simulink model "UAV_log"  (R2019b)
settings: Solver=FixedStepAuto  StartTime=0.0  StopTime=100  RelTol=1e-3
InitFcn:
  | load('BusDefinitions.mat')
values from neighbouring files (symbols this model uses):
  A_double = [0 1; 0 0]    [kalman_matrices_calculator.m]
  A_s_double = eval(subs(Ad_double,Ts))    [kalman_matrices_calculator.m]
  A_s_single = eval(subs(Ad_single,Ts))    [kalman_matrices_calculator.m]
  A_single = [0]    [kalman_matrices_calculator.m]
  B_double = [0; 1]    [kalman_matrices_calculator.m]
  B_s_double = eval(subs(Bd_double,Ts))    [kalman_matrices_calculator.m]
  B_s_single = eval(subs(Bd_single,Ts))    [kalman_matrices_calculator.m]
  B_single = [1]    [kalman_matrices_calculator.m]
  C_double = [1 0]    [kalman_matrices_calculator.m]
  C_single = [1]    [kalman_matrices_calculator.m]
  D_double = [0]    [kalman_matrices_calculator.m]
  D_single = [0]    [kalman_matrices_calculator.m]
  L_double = lqe(A_double, G_double, C_double, q_double, r_double, 0)    [kalman_matrices_calculator.m]
  L_single = lqe(A_single, G_single, C_single, q_single, r_single, 0)    [kalman_matrices_calculator.m]
  q_single = cov(out.In_Out_Data{1}.Values.Data)    [kalman_matrices_calculator.m]
  r_single = cov(out.In_Out_Data{2}.Values.Data)    [kalman_matrices_calculator.m]
  Ts = 0.005    [kalman_matrices_calculator.m]
undefined symbols (not defined in the file or in its folder): codertarget, DiscIntNeverNeededParam, Discrete, Time
libraries: ctrlSharedLib x5
settings Model: ExtModeTrigDuration=80  Creator=Sankalp Bhan  LastModifiedBy=Chris
settings OptimizationCC: PassReuseOutputArgsThreshold=0  MaxStackSize=64
settings DebuggingCC: ParameterTunabilityLossMsg=error  ArithmeticOperatorsInVariantConditions=warning
settings HardwareCC: ProdBitPerPointer=32  ProdBitPerSizeT=32  ProdBitPerPtrDiffT=32  ProdLargestAtomicInteger=Long  ProdWordSize=32  ProdHWDeviceType=ARM Compatible->ARM 9  UseEmbeddedCoderFeatures=off
settings SFSimCC: SimUseLocalCustomCode=off  MATLABDynamicMemAlloc=off
settings RTWCC: SystemTargetFile=ert.tlc  HardwareBoard=PARROT Mambo  TLCOptions="-aInlineSetEventsForThisBaseRateFcn=TLC_FALSE -aSuppressMultiTaskScheduler=TLC_FALSE   -aRateBasedStepFcn=1"  TemplateMakefile=ert_default_tmf  GenerateReport=on  RTWUseLocalCustomCode=off  Toolchain=Sourcery G++ Lite GNU Toolchain for Drones  LaunchReport=on
settings CodeAppCC: ForceParamTrailComments=on  OperatorAnnotations=on  StateflowObjectComments=on
settings ERTTargetCC: ERTCustomFileBanners=off  MatFileLogging=on  SupportContinuousTime=on  SupportNonInlinedSFcns=on  RemoveResetFunc=off  ModelStepFunctionPrototypeControlCompliant=off

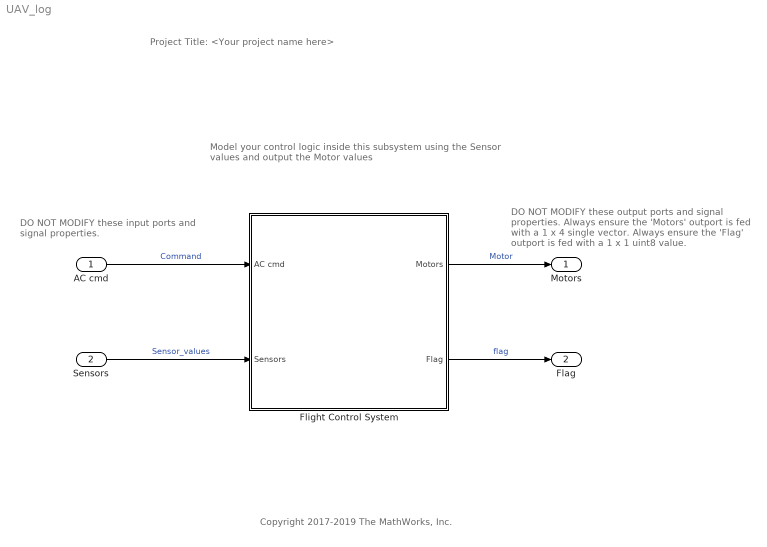
== system UAV_log ==
  note: Model your control logic inside this subsystem
      | using the Sensor values and output the
      | Motor values
  note: DO NOT MODIFY these output ports
      | and signal properties.
      |
      |
      |
      | Always ensure the 'Motors' outport
      | is fed with a 1 x 4 single vector.
      |
      |
      |
      |
      |
      | Always ensure the 'Flag' outport is
      | fed with a 1 x 1 uint8 value.
  note: DO NOT MODIFY these input
      | ports and signal properties.
  note: Copyright 2017-2019 The MathWorks, Inc.
  note: Project Title: <Your project name here>
  AC cmd : Inport  OutDataTypeStr=Bus: CommandBus  BusOutputAsStruct=on
  Sensors : Inport  Port=2  OutDataTypeStr=Bus: SensorsBus  BusOutputAsStruct=on
  Flight Control System : Subsystem  InitFcn=codertarget.parrot.internal.fcsSubsystemCallback(gcb);
  Motors : Outport  OutDataTypeStr=single  PortDimensions=[1 4]  VectorParamsAs1DForOutWhenUnconnected=off
  Flag : Outport  Port=2  OutDataTypeStr=uint8  PortDimensions=1  VectorParamsAs1DForOutWhenUnconnected=off
  wires:
  Flight Control System/1(Motors) -> Motors/1  "Motor"
  AC cmd/1 -> Flight Control System/1(AC cmd)  "Command"
  Sensors/1 -> Flight Control System/2(Sensors)  "Sensor_values"
  Flight Control System/2(Flag) -> Flag/1  "flag"

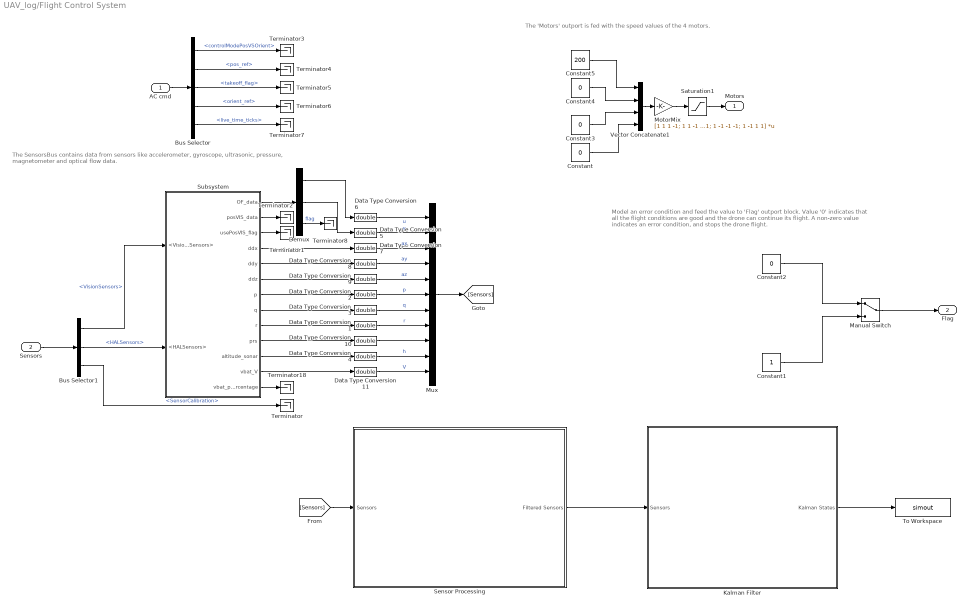
== system UAV_log/Flight Control System ==
  note: The 'Motors' outport is fed with the speed values of the 4 motors.
  note: Model an error condition and feed the value to 'Flag' outport block.
      | Value '0' indicates that all the flight conditions are good and the drone
      | can continue its flight.
      | A non-zero value indicates an error condition, and stops the drone
      | flight.
  note: The SensorsBus contains data from sensors like
      | accelerometer, gyroscope, ultrasonic, pressure,
      | magnetometer and optical flow data.
  AC cmd : Inport
  Sensors : Inport  Port=2
  Bus Selector : BusSelector  OutputSignals=controlModePosVSOrient,pos_ref,takeoff_flag,orient_ref,live_time_ticks
  Bus Selector1 : BusSelector  OutputSignals=VisionSensors,HALSensors,SensorCalibration
  Constant : Constant  Value=0  SampleTime=Ts
  Constant1 : Constant  OutDataTypeStr=uint8
  Constant2 : Constant  Value=0  OutDataTypeStr=uint8
  Constant3 : Constant  Value=0  SampleTime=Ts
  Constant4 : Constant  Value=0  SampleTime=Ts
  Constant5 : Constant  Value=200  SampleTime=Ts
  Data Type Conversion{1..11} (11 alike) : DataTypeConversion  OutDataTypeStr=double
  Demux : Demux  Outputs=3
  Kalman Filter : Subsystem
  Manual Switch : ManualSwitch
  MotorMix : Gain  Gain=[1 1 1 -1; 1 1 -1 1; 1 -1 -1 -1; 1 -1 1 1]  Multiplication=Matrix(K*u)
  Mux : Mux  Inputs=11
  Saturation1 : Saturate  UpperLimit=500  LowerLimit=0  OutDataTypeStr=single
  "Sensor Processing " : Subsystem
  Subsystem : Subsystem
  Terminator{,1..8,18} (10 alike) : Terminator
  To Workspace : ToWorkspace  VariableName=simout  SaveFormat=Structure With Time  SampleTime=-1
  Vector Concatenate1 : Concatenate  NumInputs=4
  Motors : Outport  VectorParamsAs1DForOutWhenUnconnected=off
  Flag : Outport  Port=2  VectorParamsAs1DForOutWhenUnconnected=off
  wires:
  AC cmd/1 -> Bus Selector/1
  Sensors/1 -> Bus Selector1/1
  Bus Selector/1 -> Terminator3/1  "<controlModePosVSOrient>"
  Bus Selector/2 -> Terminator4/1  "<pos_ref>"
  Bus Selector/3 -> Terminator5/1  "<takeoff_flag>"
  Bus Selector/4 -> Terminator6/1  "<orient_ref>"
  Bus Selector/5 -> Terminator7/1  "<live_time_ticks>"
  Manual Switch/1 -> Flag/1
  Constant2/1 -> Manual Switch/1
  Constant1/1 -> Manual Switch/2
  Vector Concatenate1/1 -> MotorMix/1
  Constant5/1 -> Vector Concatenate1/1
  Constant/1 -> Vector Concatenate1/4
  Constant4/1 -> Vector Concatenate1/2
  Constant3/1 -> Vector Concatenate1/3
  Saturation1/1 -> Motors/1
  Bus Selector1/1 -> Subsystem/1(<VisionSensors>)  "<VisionSensors>"
  Bus Selector1/2 -> Subsystem/2(<HALSensors>)  "<HALSensors>"
  Bus Selector1/3 -> Terminator/1  "<SensorCalibration>"
  Subsystem/1(OF_data) -> Demux/1
  Subsystem/4(ddx) -> Data Type Conversion7/1
  Subsystem/5(ddy) -> Data Type Conversion8/1
  Subsystem/6(ddz) -> Data Type Conversion9/1
  Subsystem/7(p) -> Data Type Conversion2/1
  Subsystem/9(r) -> Data Type Conversion1/1
  Subsystem/11(altitude_sonar) -> Data Type Conversion4/1
  Subsystem/12(vbat_V) -> Data Type Conversion11/1
  Subsystem/13(vbat_percentage) -> Terminator18/1
  Subsystem/8(q) -> Data Type Conversion3/1
  Mux/1 -> [Sensors]
  MotorMix/1 -> Saturation1/1
  Subsystem/3(usePosVIS_flag) -> Terminator1/1
  Subsystem/2(posVIS_data) -> Terminator2/1
  Demux/1 -> Data Type Conversion6/1
  Demux/2 -> Data Type Conversion5/1
  Demux/3 -> Terminator8/1  "flag"
  Subsystem/10(prs) -> Data Type Conversion10/1
  Data Type Conversion1/1 -> Mux/8  "r"
  Data Type Conversion2/1 -> Mux/6  "p"
  Data Type Conversion3/1 -> Mux/7  "q"
  Data Type Conversion4/1 -> Mux/10  "h"
  Data Type Conversion5/1 -> Mux/2  "v"
  Data Type Conversion6/1 -> Mux/1  "u"
  Data Type Conversion7/1 -> Mux/3  "ax"
  Data Type Conversion8/1 -> Mux/4  "ay"
  Data Type Conversion9/1 -> Mux/5  "az"
  Data Type Conversion10/1 -> Mux/9
  Data Type Conversion11/1 -> Mux/11  "V"
  [Sensors] -> "Sensor Processing "/1(Sensors)
  "Sensor Processing "/1(Filtered Sensors) -> Kalman Filter/1(Sensors)
  Kalman Filter/1(Kalman States) -> To Workspace/1

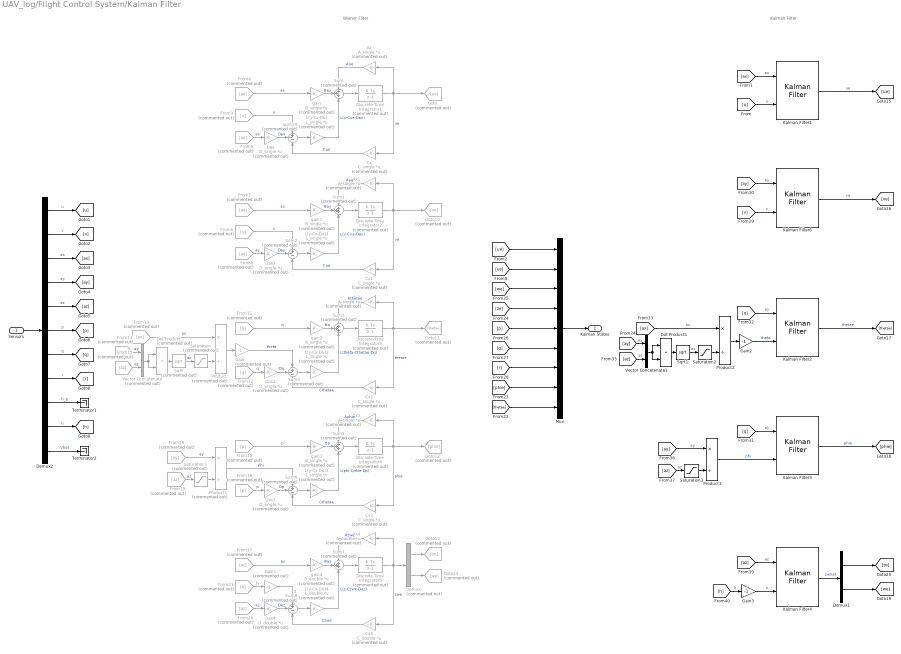
== system UAV_log/Flight Control System/Kalman Filter ==
  note: Wiener Filter
  note: Kalman Filter
  Sensors : Inport
  Ax{,1..3} (4 alike) : Gain  Commented=on  Gain=A_single  Multiplication=Matrix(K*u)
      settings: AttributesFormatString=Ax
  Ax4 : Gain  Commented=on  Gain=A_double  Multiplication=Matrix(K*u)
      settings: AttributesFormatString=Ax
  Cx{,1..3} (4 alike) : Gain  Commented=on  Gain=C_single  Multiplication=Matrix(K*u)
      settings: AttributesFormatString=Cx
  Cx4 : Gain  Commented=on  Gain=C_double  Multiplication=Matrix(K*u)
      settings: AttributesFormatString=Cx
  Dax{,1..3} (4 alike) : Gain  Commented=on  Gain=D_single  Multiplication=Matrix(K*u)
      settings: AttributesFormatString=Du
  Dax4 : Gain  Commented=on  Gain=D_double  Multiplication=Matrix(K*u)
      settings: AttributesFormatString=Du
  Demux : Demux  Commented=on  Outputs=2
  Demux1 : Demux  Outputs=2
  Demux2 : Demux  Outputs=11
  Discrete-Time Integrator{1..5} (5 alike) : DiscreteIntegrator  Commented=on  SampleTime=-1  ICPrevOutput=DiscIntNeverNeededParam  ICPrevScaledInput=DiscIntNeverNeededParam
  Dot Product : DotProduct  Commented=on  OutMin=0.0001  InputSameDT=on  OutDataTypeStr=Inherit: Inherit via internal rule
  Dot Product1 : DotProduct  OutMin=0.0001  InputSameDT=on  OutDataTypeStr=Inherit: Inherit via internal rule
  From10 : From  Commented=on  GotoTag=p
  From11 : From  Commented=on  GotoTag=q
  From12 : From  Commented=on  GotoTag=q
  From13 : From  Commented=on  GotoTag=ax
  From{7..8,14,18} (4 alike) : From  Commented=on  GotoTag=ay
  From{15,17,19..20} (4 alike) : From  Commented=on  GotoTag=az
  From16 : From  Commented=on  GotoTag=p
  From21 : From  Commented=on  GotoTag=h
  From3 : From  Commented=on  GotoTag=u
  From4 : From  Commented=on  GotoTag=ax
  From5 : From  Commented=on  GotoTag=ax
  From6 : From  Commented=on  GotoTag=v
  Gain : Gain  Commented=on  Gain=-1
  Gain1 : Gain  Commented=on  Gain=-1
  Gain2 : Gain  Gain=-1
  Gain3 : Gain  Gain=-1
  Goto : Goto  Commented=on  GotoTag=ue
  Goto10 : Goto  Commented=on  GotoTag=ve
  Goto11 : Goto  Commented=on  GotoTag=thetae
  Goto12 : Goto  Commented=on  GotoTag=phie
  Goto13 : Goto  Commented=on  GotoTag=we
  Goto14 : Goto  Commented=on  GotoTag=ze
  Kalman Filter{1..3,6} (4 alike) : ctrlSharedLib/Kalman Filter  TimeDomain=Discrete-Time  UseCurrentEstimator=on  ModelSource=Individual A, B, C, D matrices  ModelSourceVariable=ss(0.95,1,1,0,1)  A=A_s_single  B=B_s_single  C=C_single  D=D_single  NumberOfStates=1  NumberOfInputs=1  NumberOfOutputs=1  InitialEstimateSource=Dialog  X0=[0]  P0=10  UseK=off  UseGH=off  NumberOfProcessNoiseInputs=1  G=1  TimeInvariantG=on  H=0  TimeInvariantH=on  Q=[1]*q_single  TimeInvariantQ=on  R=[1]*r_single*10000  TimeInvariantR=on  N=0  TimeInvariantN=on  AddInputPort=on  AddEnablePort=off  OutputEstimatedY=off  OutputP=off  Ts=Ts
      settings: SourceProductBaseCode=CT
  Kalman Filter4 : ctrlSharedLib/Kalman Filter  TimeDomain=Discrete-Time  UseCurrentEstimator=on  ModelSource=Individual A, B, C, D matrices  ModelSourceVariable=ss(0.95,1,1,0,1)  A=A_s_double  B=B_s_double  C=C_double  D=D_double  NumberOfStates=1  NumberOfInputs=1  NumberOfOutputs=1  InitialEstimateSource=Dialog  X0=[0]  P0=10  UseK=off  UseGH=off  NumberOfProcessNoiseInputs=1  G=1  TimeInvariantG=on  H=0  TimeInvariantH=on  Q=[1]*q_single  TimeInvariantQ=on  R=[1]*r_single*10000  TimeInvariantR=on  N=0  TimeInvariantN=on  AddInputPort=on  AddEnablePort=off  OutputEstimatedY=off  OutputP=off  Ts=Ts
      settings: SourceProductBaseCode=CT
  L(y-Cx-Du){,1..3} (4 alike) : Gain  Commented=on  Gain=L_single  Multiplication=Matrix(K*u)
      settings: AttributesFormatString=L(y-Cx-Du)
  L(y-Cx-Du)4 : Gain  Commented=on  Gain=L_double  Multiplication=Matrix(K*u)
      settings: AttributesFormatString=L(y-Cx-Du)
  Mux : Mux  Inputs=9
  Product : Product  Commented=on  Inputs=*/
  Product1 : Product  Commented=on  Inputs=*/
  Product2 : Product  Inputs=*/
  Product3 : Product  Inputs=*/
  Saturation : Saturate  Commented=on  UpperLimit=inf  LowerLimit=0.001
  Saturation1 : Saturate  Commented=on  UpperLimit=inf  LowerLimit=0.001
  Saturation2 : Saturate  UpperLimit=inf  LowerLimit=0.001
  Saturation3 : Saturate  UpperLimit=inf  LowerLimit=0.001
  Sqrt : Sqrt  Commented=on  SaturateOnIntegerOverflow=on
  Sqrt1 : Sqrt  SaturateOnIntegerOverflow=on
  Sum{,1,3,5,7} (5 alike) : Sum  Commented=on  Inputs=+++
  Sum{2,4,6,8,10} (5 alike) : Sum  Commented=on  Inputs=+--
  Terminator1 : Terminator
  Terminator2 : Terminator
  Vector Concatenate : Concatenate  Commented=on
  Vector Concatenate1 : Concatenate
  gain{,1..3} (4 alike) : Gain  Commented=on  Gain=B_single  Multiplication=Matrix(K*u)
      settings: AttributesFormatString=Bu
  gain4 : Gain  Commented=on  Gain=B_double  Multiplication=Matrix(K*u)
      settings: AttributesFormatString=Bu
  Kalman States : Outport
  wires:
  Discrete-Time Integrator1/1 -> Goto/1, Cx/1, Ax/1  "ue"
  Sum10/1 -> L(y-Cx-Du)/1
  Ax/1 -> Sum/1  "Aue"
  L(y-Cx-Du)/1 -> Sum/3  "L(u-Cue-Dax)"
  Cx/1 -> Sum10/3  "Cue"
  From4/1 -> gain/1  "ax"
  gain/1 -> Sum/2  "Bax"
  From3/1 -> Sum10/1  "u"
  From5/1 -> Dax/1  "ax"
  Dax/1 -> Sum10/2  "Dax"
  Sum/1 -> Discrete-Time Integrator1/1
  Demux2/9 -> Terminator1/1  "h_p"
  Demux2/1 -> [u]  "u"
  Demux2/4 -> [ay]  "ay"
  Demux2/3 -> [ax]  "ax"
  Sensors/1 -> Demux2/1
  Demux2/2 -> [v]  "v"
  Demux2/10 -> [h]  "h"
  Demux2/5 -> [az]  "az"
  Demux2/7 -> [q]  "q"
  Demux2/8 -> [r]  "r"
  Demux2/6 -> [p]  "p"
  Demux2/11 -> Terminator2/1  "Vbat"
  Sum1/1 -> Discrete-Time Integrator2/1
  Dax1/1 -> Sum2/2  "Day"
  From8/1 -> Dax1/1  "ay"
  From6/1 -> Sum2/1  "u"
  gain1/1 -> Sum1/2  "Bay"
  From7/1 -> gain1/1  "ax"
  Cx1/1 -> Sum2/3  "Cue"
  L(y-Cx-Du)1/1 -> Sum1/3  "L(v-Cve-Day)"
  Ax1/1 -> Sum1/1  "Aue"
  Sum2/1 -> L(y-Cx-Du)1/1
  Discrete-Time Integrator2/1 -> Ax1/1, Cx1/1, Goto10/1  "ve"
  Discrete-Time Integrator3/1 -> Goto11/1, Cx2/1, Ax2/1  "thetae"
  Sum4/1 -> L(y-Cx-Du)2/1
  Ax2/1 -> Sum3/1  "Athetae"
  L(y-Cx-Du)2/1 -> Sum3/3  "L(theta-Cthetae-Dq)"
  Cx2/1 -> Sum4/3  "Cthetae"
  From11/1 -> gain2/1  "q"
  gain2/1 -> Sum3/2  "Bq"
  Gain/1 -> Sum4/1  "theta"
  From12/1 -> Dax2/1  "q"
  Dax2/1 -> Sum4/2  "Dq"
  Sum3/1 -> Discrete-Time Integrator3/1
  From14/1 -> Vector Concatenate/1  "ay"
  From15/1 -> Vector Concatenate/2  "az"
  Vector Concatenate/1 -> Dot Product/1, Dot Product/2
  Dot Product/1 -> Sqrt/1
  From13/1 -> Product/1  "ax"
  Product/1 -> Gain/1
  From18/1 -> Product1/1  "ay"
  Sum5/1 -> Discrete-Time Integrator4/1
  Dax3/1 -> Sum6/2  "Dp"
  From16/1 -> Dax3/1  "p"
  Product1/1 -> Sum6/1  "phi"
  gain3/1 -> Sum5/2  "Bp"
  From10/1 -> gain3/1  "p"
  Cx3/1 -> Sum6/3  "Cthetae"
  L(y-Cx-Du)3/1 -> Sum5/3  "L(phi-Cphie-Dp)"
  Ax3/1 -> Sum5/1  "Aphie"
  Sum6/1 -> L(y-Cx-Du)3/1
  Discrete-Time Integrator4/1 -> Ax3/1, Cx3/1, Goto12/1  "phie"
  Discrete-Time Integrator5/1 -> Ax4/1, Demux/1, Cx4/1  "zwe"
  Sum8/1 -> L(y-Cx-Du)4/1
  Ax4/1 -> Sum7/1  "Azwe"
  L(y-Cx-Du)4/1 -> Sum7/3  "L(z-Czwe-Daz)"
  Cx4/1 -> Sum8/3  "Czwe"
  From17/1 -> gain4/1  "az"
  gain4/1 -> Sum7/2  "Baz"
  From21/1 -> Gain1/1  "h"
  From20/1 -> Dax4/1  "az"
  Dax4/1 -> Sum8/2  "Daz"
  Sum7/1 -> Discrete-Time Integrator5/1
  Demux/2 -> Goto13/1
  Demux/1 -> Goto14/1
  Gain1/1 -> Sum8/1  "z"
  [ue] -> Mux/1
  [ve] -> Mux/2
  [we] -> Mux/3
  [ze] -> Mux/4
  Mux/1 -> Kalman States/1
  [r] -> Mux/7
  [q] -> Mux/6
  [p] -> Mux/5
  [phie] -> Mux/8
  [thetae] -> Mux/9
  [ax] -> Kalman Filter1/1  "ax"
  [u] -> Kalman Filter1/2  "u"
  [v] -> Kalman Filter6/2  "v"
  [ay] -> Kalman Filter6/1  "ay"
  [q] -> Kalman Filter2/1  "ay"
  Gain2/1 -> Kalman Filter2/2  "theta"
  Sqrt/1 -> Saturation/1  "az"
  Saturation/1 -> Product/2
  From19/1 -> Saturation1/1  "az"
  Saturation1/1 -> Product1/2
  Saturation2/1 -> Product2/2
  Sqrt1/1 -> Saturation2/1  "az"
  Product2/1 -> Gain2/1
  [ax] -> Product2/1  "ax"
  Dot Product1/1 -> Sqrt1/1
  Vector Concatenate1/1 -> Dot Product1/2, Dot Product1/1
  [az] -> Vector Concatenate1/2  "az"
  [ay] -> Vector Concatenate1/1  "ay"
  [q] -> Kalman Filter3/1  "ay"
  Saturation3/1 -> Product3/2
  [az] -> Saturation3/1  "az"
  Product3/1 -> Kalman Filter3/2  "phi"
  [ay] -> Product3/1  "ay"
  Kalman Filter4/1 -> Demux1/1  "zwhat"
  [az] -> Kalman Filter4/1  "az"
  Gain3/1 -> Kalman Filter4/2  "z"
  Demux1/1 -> [ze]
  Demux1/2 -> [we]
  Kalman Filter3/1 -> [phie]  "phie"
  Kalman Filter2/1 -> [thetae]  "thetae"
  Kalman Filter6/1 -> [ve]  "ve"
  Kalman Filter1/1 -> [ue]  "ue"
  [h] -> Gain3/1  "h"

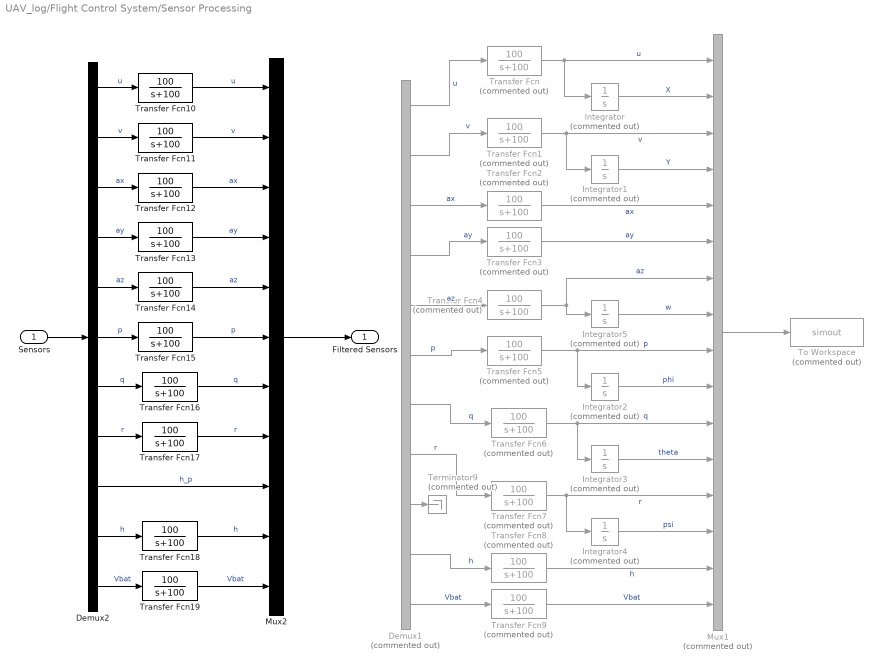
== system UAV_log/Flight Control System/Sensor Processing  ==
  Sensors : Inport
  Demux1 : Demux  Commented=on  Outputs=11
  Demux2 : Demux  Outputs=11
  Integrator{,1..5} (6 alike) : Integrator  Commented=on
  Mux1 : Mux  Commented=on  Inputs=16
  Mux2 : Mux  Inputs=11
  Terminator9 : Terminator  Commented=on
  To Workspace : ToWorkspace  Commented=on  VariableName=simout  SaveFormat=Structure With Time  SampleTime=-1
  Transfer Fcn{,1..9} (10 alike) : TransferFcn  Commented=on  Numerator=[100]  Denominator=[1 100]
  Transfer Fcn{10..19} (10 alike) : TransferFcn  Numerator=[100]  Denominator=[1 100]
  Filtered Sensors : Outport
  wires:
  Transfer Fcn2/1 -> Mux1/5  "ax"
  Integrator4/1 -> Mux1/14  "psi"
  Integrator/1 -> Mux1/2  "X"
  Integrator5/1 -> Mux1/8  "w"
  Demux1/9 -> Terminator9/1
  Demux1/5 -> Transfer Fcn4/1  "az"
  Transfer Fcn5/1 -> Integrator2/1, Mux1/9  "p"
  Transfer Fcn9/1 -> Mux1/16  "Vbat"
  Integrator2/1 -> Mux1/10  "phi"
  Demux1/7 -> Transfer Fcn6/1  "q"
  Transfer Fcn4/1 -> Integrator5/1, Mux1/7  "az"
  Demux1/10 -> Transfer Fcn8/1  "h"
  Transfer Fcn7/1 -> Mux1/13, Integrator4/1  "r"
  Integrator1/1 -> Mux1/4  "Y"
  Transfer Fcn3/1 -> Mux1/6  "ay"
  Transfer Fcn/1 -> Integrator/1, Mux1/1  "u"
  Demux1/8 -> Transfer Fcn7/1  "r"
  Transfer Fcn1/1 -> Integrator1/1, Mux1/3  "v"
  Demux1/1 -> Transfer Fcn/1  "u"
  Demux1/4 -> Transfer Fcn3/1  "ay"
  Demux1/3 -> Transfer Fcn2/1  "ax"
  Mux1/1 -> To Workspace/1
  Transfer Fcn6/1 -> Integrator3/1, Mux1/11  "q"
  Demux1/6 -> Transfer Fcn5/1  "p"
  Demux1/11 -> Transfer Fcn9/1  "Vbat"
  Transfer Fcn8/1 -> Mux1/15  "h"
  Demux1/2 -> Transfer Fcn1/1  "v"
  Integrator3/1 -> Mux1/12  "theta"
  Mux2/1 -> Filtered Sensors/1
  Demux2/2 -> Transfer Fcn11/1  "v"
  Transfer Fcn18/1 -> Mux2/10  "h"
  Demux2/11 -> Transfer Fcn19/1  "Vbat"
  Sensors/1 -> Demux2/1
  Demux2/6 -> Transfer Fcn15/1  "p"
  Transfer Fcn16/1 -> Mux2/7  "q"
  Demux2/3 -> Transfer Fcn12/1  "ax"
  Demux2/4 -> Transfer Fcn13/1  "ay"
  Demux2/1 -> Transfer Fcn10/1  "u"
  Transfer Fcn11/1 -> Mux2/2  "v"
  Demux2/8 -> Transfer Fcn17/1  "r"
  Transfer Fcn10/1 -> Mux2/1  "u"
  Transfer Fcn13/1 -> Mux2/4  "ay"
  Transfer Fcn17/1 -> Mux2/8  "r"
  Demux2/10 -> Transfer Fcn18/1  "h"
  Transfer Fcn14/1 -> Mux2/5  "az"
  Demux2/7 -> Transfer Fcn16/1  "q"
  Transfer Fcn19/1 -> Mux2/11  "Vbat"
  Transfer Fcn15/1 -> Mux2/6  "p"
  Demux2/5 -> Transfer Fcn14/1  "az"
  Demux2/9 -> Mux2/9  "h_p"
  Transfer Fcn12/1 -> Mux2/3  "ax"

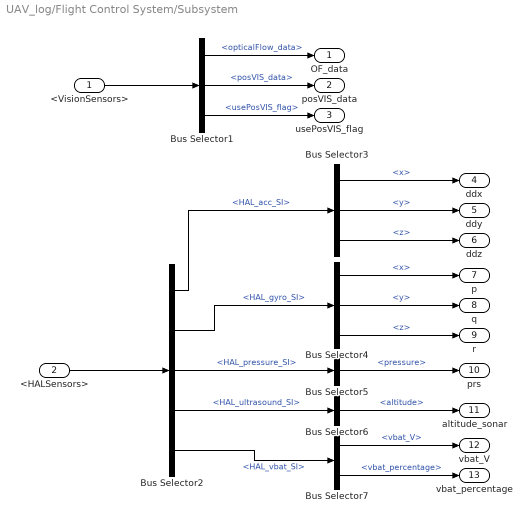
== system UAV_log/Flight Control System/Subsystem ==
  <VisionSensors> : Inport
  <HALSensors> : Inport  Port=2
  Bus Selector1 : BusSelector  OutputSignals=opticalFlow_data,posVIS_data,usePosVIS_flag
  Bus Selector2 : BusSelector  OutputSignals=HAL_acc_SI,HAL_gyro_SI,HAL_pressure_SI,HAL_ultrasound_SI,HAL_vbat_SI
  Bus Selector3 : BusSelector  OutputSignals=x,y,z
  Bus Selector4 : BusSelector  OutputSignals=x,y,z
  Bus Selector5 : BusSelector  OutputSignals=pressure
  Bus Selector6 : BusSelector  OutputSignals=altitude
  Bus Selector7 : BusSelector  OutputSignals=vbat_V,vbat_percentage
  OF_data : Outport  VectorParamsAs1DForOutWhenUnconnected=off
  posVIS_data : Outport  Port=2  VectorParamsAs1DForOutWhenUnconnected=off
  usePosVIS_flag : Outport  Port=3  VectorParamsAs1DForOutWhenUnconnected=off
  ddx : Outport  Port=4  VectorParamsAs1DForOutWhenUnconnected=off
  ddy : Outport  Port=5  VectorParamsAs1DForOutWhenUnconnected=off
  ddz : Outport  Port=6  VectorParamsAs1DForOutWhenUnconnected=off
  p : Outport  Port=7  VectorParamsAs1DForOutWhenUnconnected=off
  q : Outport  Port=8  VectorParamsAs1DForOutWhenUnconnected=off
  r : Outport  Port=9  VectorParamsAs1DForOutWhenUnconnected=off
  prs : Outport  Port=10  VectorParamsAs1DForOutWhenUnconnected=off
  altitude_sonar : Outport  Port=11  VectorParamsAs1DForOutWhenUnconnected=off
  vbat_V : Outport  Port=12  VectorParamsAs1DForOutWhenUnconnected=off
  vbat_percentage : Outport  Port=13  VectorParamsAs1DForOutWhenUnconnected=off
  wires:
  <VisionSensors>/1 -> Bus Selector1/1
  <HALSensors>/1 -> Bus Selector2/1
  Bus Selector1/1 -> OF_data/1  "<opticalFlow_data>"
  Bus Selector1/2 -> posVIS_data/1  "<posVIS_data>"
  Bus Selector1/3 -> usePosVIS_flag/1  "<usePosVIS_flag>"
  Bus Selector2/1 -> Bus Selector3/1  "<HAL_acc_SI>"
  Bus Selector2/2 -> Bus Selector4/1  "<HAL_gyro_SI>"
  Bus Selector2/3 -> Bus Selector5/1  "<HAL_pressure_SI>"
  Bus Selector2/4 -> Bus Selector6/1  "<HAL_ultrasound_SI>"
  Bus Selector2/5 -> Bus Selector7/1  "<HAL_vbat_SI>"
  Bus Selector3/1 -> ddx/1  "<x>"
  Bus Selector3/2 -> ddy/1  "<y>"
  Bus Selector3/3 -> ddz/1  "<z>"
  Bus Selector4/2 -> q/1  "<y>"
  Bus Selector4/1 -> p/1  "<x>"
  Bus Selector4/3 -> r/1  "<z>"
  Bus Selector5/1 -> prs/1  "<pressure>"
  Bus Selector6/1 -> altitude_sonar/1  "<altitude>"
  Bus Selector7/1 -> vbat_V/1  "<vbat_V>"
  Bus Selector7/2 -> vbat_percentage/1  "<vbat_percentage>"
